simulink model "Q3_sim"  (R2021a)
settings: Solver=VariableStepAuto  StartTime=0.0  StopTime=10  RelTol=1e-3
values from neighbouring files (symbols this model uses):
  A = [-1.7,-0.25,0;23,-30,20;0,-200-290,-220-920]    [Q1_code.m]    (also in Q2_code.m; Q3_code.m; Q4_code.m; Q5_code.m)
  B = [3+2,0;-30-53,0;0,-420-350]    [Q1_code.m]    (also in Q2_code.m; Q3_code.m; Q4_code.m; Q5_code.m)
  C = [0,1,0;0,0,1]    [Q1_code.m]    (also in Q2_code.m; Q3_code.m; Q4_code.m; Q5_code.m)
  C1 = eye(3)    [Q1_code.m]    (also in Q2_code.m; Q3_code.m; Q4_code.m)
  d = -3    [Q3_code.m]
  D1 = zeros(3,2)    [Q1_code.m]    (also in Q2_code.m; Q3_code.m; Q4_code.m)
  E = T*B    [Q3_code.m]
  G = [10,20]    [Q3_code.m]
  K = Kba*T    [Q1_code.m]    (also in Q2_code.m = R\B'*P; Q3_code.m = R\B'*P; Q4_code.m = B_s\C_ss; Q5_code.m = R\Bbar'*P)
  x0 = [1;100;200]    [Q1_code.m]    (also in Q2_code.m; Q3_code.m; Q4_code.m; Q5_code.m)
  zeta = 0.6    [Q1_code.m]    (also in Q3_code.m = inv([C;T]))
settings Model: Creator=l_w_h  LastModifiedBy=l_w_h

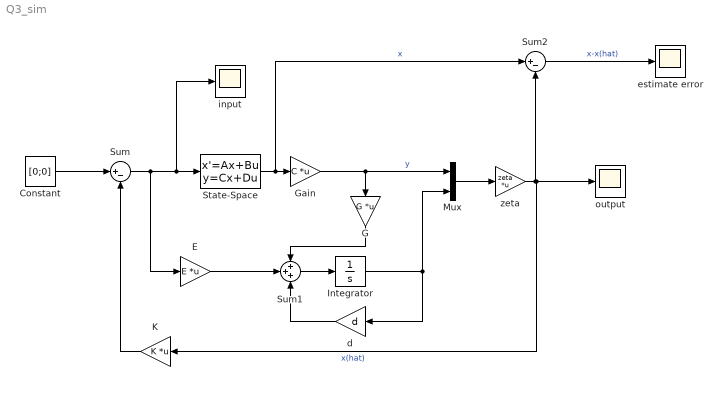
== system Q3_sim ==
  Constant : Constant  Value=[0;0]
  E : Gain  Gain=E  Multiplication=Matrix(K*u)
  G : Gain  Gain=G  Multiplication=Matrix(K*u)
  Gain : Gain  Gain=C  Multiplication=Matrix(K*u)
  Integrator : Integrator
  K : Gain  Gain=K  Multiplication=Matrix(K*u)
  Mux : Mux  Inputs=2
  State-Space : StateSpace  A=A  B=B  C=C1  D=D1  InitialCondition=x0
  Sum : Sum  Inputs=|+-
  Sum1 : Sum  Inputs=+++
  Sum2 : Sum  Inputs=|+-
  d : Gain  Gain=d
  estimate error : Scope
  input : Scope
  output : Scope
  zeta : Gain  Gain=zeta  Multiplication=Matrix(K*u)
  wires:
  State-Space/1 -> Sum2/1, Gain/1  "x"
  K/1 -> Sum/2
  Sum/1 -> E/1, input/1, State-Space/1
  Constant/1 -> Sum/1
  Gain/1 -> Mux/1, G/1  "y"
  G/1 -> Sum1/1
  E/1 -> Sum1/2
  d/1 -> Sum1/3
  Sum1/1 -> Integrator/1
  Integrator/1 -> d/1, Mux/2
  Mux/1 -> zeta/1
  zeta/1 -> output/1, K/1, Sum2/2  "x(hat)"
  Sum2/1 -> estimate error/1  "x-x(hat)"
